simulink model "SimulinkTP2"  (R2018b)
settings: Solver=VariableStepAuto  StartTime=0.0  StopTime=0.0025  RelTol=1e-3
libraries: fl_lib x13, nesl_utility x5
settings Model: Creator=A47521  LastModifiedBy=A47521

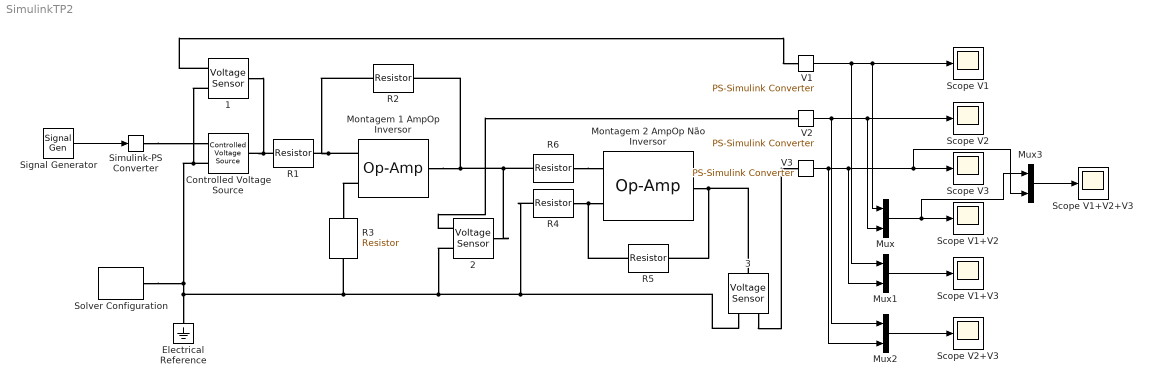
== system SimulinkTP2 ==
  1 : fl_lib/Electrical/Electrical Sensors/Voltage Sensor
  2 : fl_lib/Electrical/Electrical Sensors/Voltage Sensor
  3 : fl_lib/Electrical/Electrical Sensors/Voltage Sensor
  Controlled Voltage Source : fl_lib/Electrical/Electrical Sources/Controlled Voltage Source
  Electrical Reference : fl_lib/Electrical/Electrical Elements/Electrical Reference
  Montagem 1 AmpOp Inversor : fl_lib/Electrical/Electrical Elements/Op-Amp  outI_specify=off  outI_priority=None  outI=0 A  outI_nominal_specify=off  outI_nominal_unit=A  outI_nominal_value=1
  Montagem 2 AmpOp Não Inversor : fl_lib/Electrical/Electrical Elements/Op-Amp  outI_specify=off  outI_priority=None  outI=0 A  outI_nominal_specify=off  outI_nominal_unit=A  outI_nominal_value=1
  Mux{,1..3} (4 alike) : Mux  Inputs=2
  R{1,3..4,6} (4 alike) : fl_lib/Electrical/Electrical Elements/Resistor  R=1 kOhm  i_specify=off  i_priority=None  i=0 A  i_nominal_specify=off  i_nominal_unit=A  i_nominal_value=1  v_specify=off  v_priority=None  v=0 V  v_nominal_specify=off  v_nominal_unit=V  v_nominal_value=1
  R2 : fl_lib/Electrical/Electrical Elements/Resistor  R=4.7 kOhm  i_specify=off  i_priority=None  i=0 A  i_nominal_specify=off  i_nominal_unit=A  i_nominal_value=1  v_specify=off  v_priority=None  v=0 V  v_nominal_specify=off  v_nominal_unit=V  v_nominal_value=1
  R5 : fl_lib/Electrical/Electrical Elements/Resistor  R=4.7 kOhm  i_specify=off  i_priority=None  i=0 A  i_nominal_specify=off  i_nominal_unit=A  i_nominal_value=1  v_specify=off  v_priority=None  v=0 V  v_nominal_specify=off  v_nominal_unit=V  v_nominal_value=1
  Scope V1 : Scope
  Scope V1+V2 : Scope
  Scope V1+V2+V3 : Scope
  Scope V1+V3 : Scope
  Scope V2 : Scope
  Scope V2+V3 : Scope
  Scope V3 : Scope
  Signal Generator : SignalGenerator  Amplitude=0.2  Frequency=1000
  Simulink-PS Converter : nesl_utility/Simulink-PS Converter  PhysicalDomain=network_engine_domain  SubClassName=ps_input  LeftPortType=input  RightPortType=output  PseudoPeriodic=off  Frequencies=[]  NoiseDistribution=none  NoiseParameters=[]  Unit=1  AffineConversion=off  FilteringAndDerivatives=provide  SimscapeFilterOrder=1  InputFilterTimeConstant=0.001  UdotUserProvided=0
  Solver Configuration : nesl_utility/Solver Configuration  PhysicalDomain=network_engine_domain  SubClassName=solver  LeftPortType=input  RightPortType=generic  Tones=[]  Harmonics=[]  SimulateNoise=off  Profile=off  UseLocalSampling=off  EnableSwitchedLinearOptims=on  FrequencyDomain=off  UseCCode=off  RelTol=0.001  AbsTol=1e-06  MinStep=1e-09  ToWorkspace=off  RevertToSquareIcSolve=off  NumHomotopyIterations=100  PhasorMode=off  PhasorModeNumHarmonics=1  DoDC=off  ResidualTolerance=1e-09  UseLocalSolver=off  LocalSolverChoice=NE_BACKWARD_EULER_ADVANCER  LocalSolverSampleTime=0.001  DoFixedCost=off  MaxNonlinIter=3  MaxModeIter=2  LinearAlgebra=auto  EquationFormulation=NE_TIME_EF  DelaysMemoryBudget=1024  AutomaticFiltering=on  FilteringTimeConstant=0.001  PartitionStorageMethod=AS_NEEDED  PartitionMemoryBudget=1024
  V1 : nesl_utility/PS-Simulink Converter  PhysicalDomain=network_engine_domain  SubClassName=ps_output  LeftPortType=input  RightPortType=output  PseudoPeriodic=off  Frequencies=[]  Unit=1  AffineConversion=off
  V2 : nesl_utility/PS-Simulink Converter  PhysicalDomain=network_engine_domain  SubClassName=ps_output  LeftPortType=input  RightPortType=output  PseudoPeriodic=off  Frequencies=[]  Unit=1  AffineConversion=off
  V3 : nesl_utility/PS-Simulink Converter  PhysicalDomain=network_engine_domain  SubClassName=ps_output  LeftPortType=input  RightPortType=output  PseudoPeriodic=off  Frequencies=[]  Unit=1  AffineConversion=off
  wires:
  V2/1 -> Mux2/1, Scope V2/1, Mux/2
  V3/1 -> Mux2/2, Mux1/2, Scope V3/1, Mux3/2
  Signal Generator/1 -> Simulink-PS Converter/1
  Mux/1 -> Mux3/1, Scope V1+V2/1
  Mux1/1 -> Scope V1+V3/1
  Mux2/1 -> Scope V2+V3/1
  Mux3/1 -> Scope V1+V2+V3/1
  V1/1 -> Mux1/1, Mux/1, Scope V1/1
  connections:
  R4/LConn1 -- R3/RConn1 -- Electrical Reference/LConn1 -- Controlled Voltage Source/RConn2 -- 1/RConn2 -- Solver Configuration/RConn1 -- 2/RConn2 -- 3/RConn2
  R1/LConn1 -- 1/LConn1 -- Controlled Voltage Source/LConn1
  R2/LConn1 -- Montagem 1 AmpOp Inversor/LConn2 -- R1/RConn1
  Montagem 1 AmpOp Inversor/RConn1 -- R6/LConn1 -- 2/LConn1 -- R2/RConn1
  R6/RConn1 -- Montagem 2 AmpOp Não Inversor/LConn1
  R4/RConn1 -- R5/LConn1 -- Montagem 2 AmpOp Não Inversor/LConn2
  Montagem 1 AmpOp Inversor/LConn1 -- R3/LConn1
  Montagem 2 AmpOp Não Inversor/RConn1 -- R5/RConn1 -- 3/LConn1
  Simulink-PS Converter/RConn1 -- Controlled Voltage Source/RConn1
  1/RConn1 -- V1/LConn1
  2/RConn1 -- V2/LConn1
  3/RConn1 -- V3/LConn1
